simulink model "stanley"  (R2025b)
settings: Solver=VariableStepAuto  StartTime=0.0  StopTime=10.0  RelTol=1e-3
libraries: drivingvehiclecontroller x1
settings Model: Creator=hubertm  LastModifiedBy=hubertm

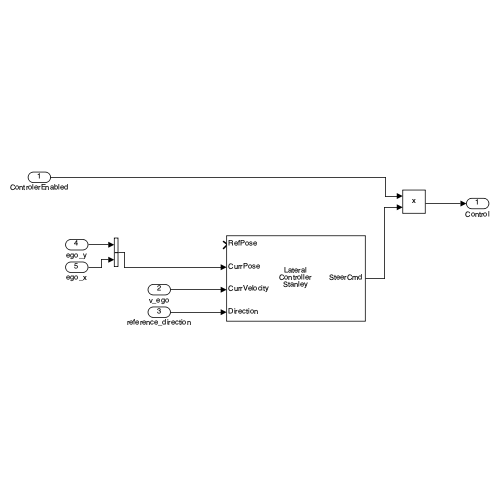
[thumbnail: Simulink's stored preview of the top-level diagram]
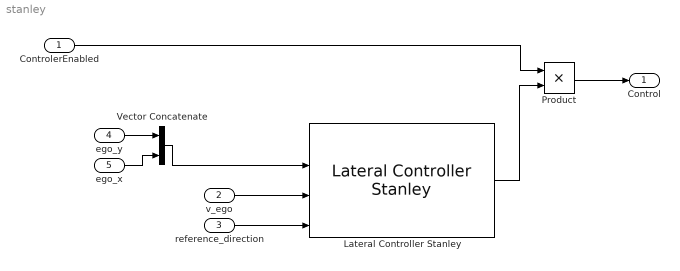
== system stanley ==
  ControlerEnabled : Inport
  v_ego : Inport  Port=2
  reference_direction : Inport  Port=3
  ego_y : Inport  Port=4
  ego_x : Inport  Port=5
  Lateral Controller Stanley : drivingvehiclecontroller/Lateral Controller Stanley  ModelType=Kinematic bicycle model  PositionGainF=2.5  PositionGainR=2.5  YawRateGain=0.2  DelayGain=0.2  VehicleMass=1575  Lf=1.2  Lr=1.6  TireStiffness=19000  Wheelbase=2.8  MaxSteeringAngle=35
  Product : Product
  Vector Concatenate : Concatenate
  Control : Outport
  wires:
  ControlerEnabled/1 -> Product/1
  Lateral Controller Stanley/1 -> Product/2
  Product/1 -> Control/1
  v_ego/1 -> Lateral Controller Stanley/3
  reference_direction/1 -> Lateral Controller Stanley/4
  ego_x/1 -> Vector Concatenate/2
  ego_y/1 -> Vector Concatenate/1
  Vector Concatenate/1 -> Lateral Controller Stanley/2
